simulink model "untitled"  (R2026a)
settings: Solver=FixedStepDiscrete  StartTime=0  StopTime=0.2  FixedStep=5e-05
settings Model: Creator=nairizeytounzian  LastModifiedBy=nairizeytounzian

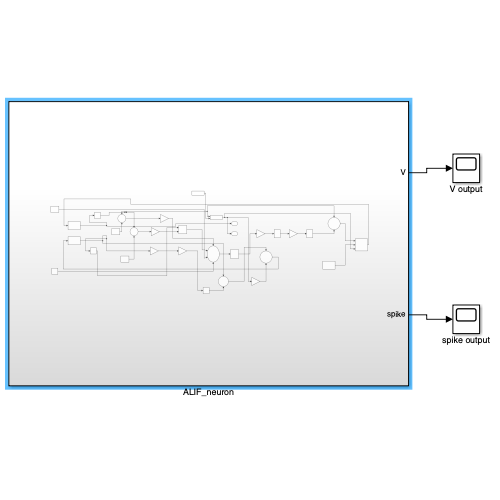
[thumbnail: Simulink's stored preview of the top-level diagram]
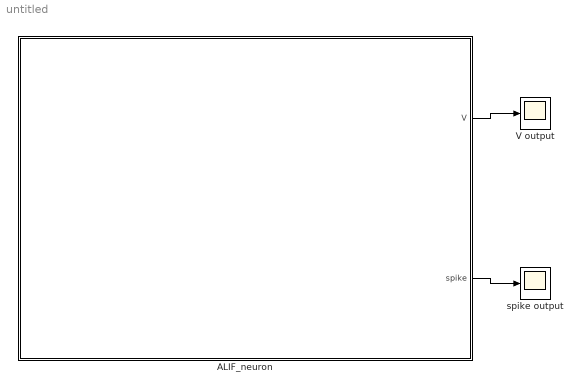
== system untitled ==
  ALIF_neuron : Subsystem
  V output : Scope
      settings: ActiveDisplayYMinimum=-74.012180112119538  ActiveDisplayYMaximum=-48.080272939355147
  spike output : Scope
      settings: ActiveDisplayYMinimum=-0.12499999999999997  ActiveDisplayYMaximum=1.125
  wires:
  ALIF_neuron/1(V) -> V output/1
  ALIF_neuron/2(spike) -> spike output/1

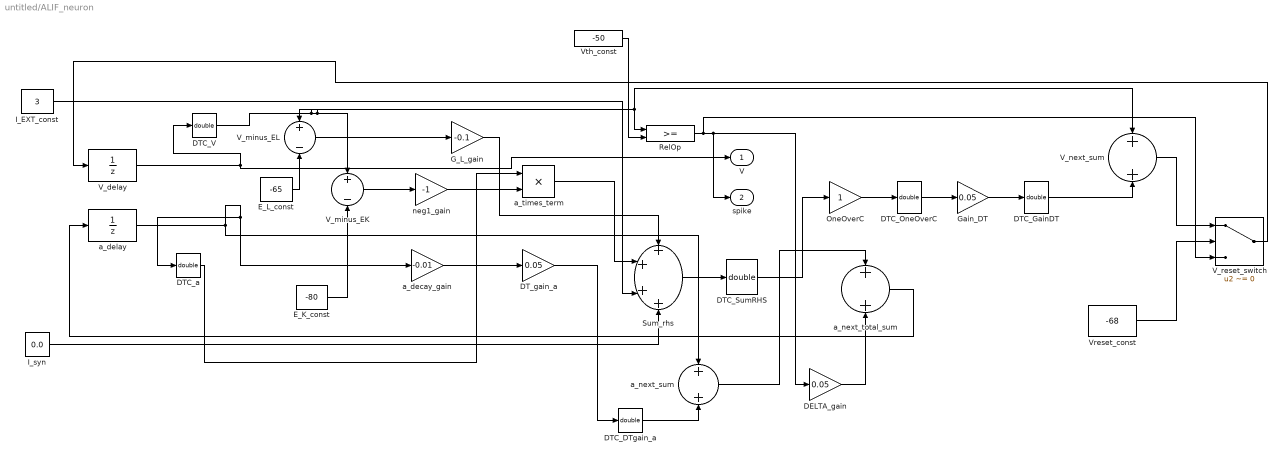
== system untitled/ALIF_neuron ==
  DELTA_gain : Gain  Gain=0.05
  DTC_DTgain_a : DataTypeConversion  OutDataTypeStr=double  SaturateOnIntegerOverflow=off  RndMeth=Floor
  DTC_GainDT : DataTypeConversion  OutDataTypeStr=double  SaturateOnIntegerOverflow=off  RndMeth=Floor
  DTC_OneOverC : DataTypeConversion  OutDataTypeStr=double  SaturateOnIntegerOverflow=off  RndMeth=Floor
  DTC_SumRHS : DataTypeConversion  OutDataTypeStr=double  SaturateOnIntegerOverflow=off  RndMeth=Floor
  DTC_V : DataTypeConversion  OutDataTypeStr=double  SaturateOnIntegerOverflow=off  RndMeth=Floor
  DTC_a : DataTypeConversion  OutDataTypeStr=double  SaturateOnIntegerOverflow=off  RndMeth=Floor
  DT_gain_a : Gain  Gain=0.05
  E_K_const : Constant  Value=-80  OutDataTypeStr=double
  E_L_const : Constant  Value=-65  OutDataTypeStr=double
  G_L_gain : Gain  Gain=-0.1
  Gain_DT : Gain  Gain=0.05
  I_EXT_const : Constant  Value=3  OutDataTypeStr=double
  I_syn : Constant  Value=0.0
  OneOverC : Gain
  RelOp : RelationalOperator  OutDataTypeStr=boolean  RndMeth=Simplest  InputSameDT=off
  Sum_rhs : Sum  Inputs=++++
  V_delay : UnitDelay  InitialCondition=-65  SampleTime=-1
  V_minus_EK : Sum  Inputs=+-
  V_minus_EL : Sum  Inputs=+-
  V_next_sum : Sum
  V_reset_switch : Switch  Criteria=u2 ~= 0  Threshold=0.5  SaturateOnIntegerOverflow=off  InputSameDT=off
  Vreset_const : Constant  Value=-68  OutDataTypeStr=double
  Vth_const : Constant  Value=-50  OutDataTypeStr=double
  a_decay_gain : Gain  Gain=-0.01
  a_delay : UnitDelay  SampleTime=-1
  a_next_sum : Sum
  a_next_total_sum : Sum
  a_times_term : Product
  neg1_gain : Gain  Gain=-1
  V : Outport
  spike : Outport  Port=2
  wires:
  V_delay/1 -> DTC_V/1, V/1
  DTC_V/1 -> V_minus_EK/1, V_minus_EL/1, V_next_sum/1, RelOp/1
  E_L_const/1 -> V_minus_EL/2
  E_K_const/1 -> V_minus_EK/2
  V_minus_EL/1 -> G_L_gain/1
  G_L_gain/1 -> Sum_rhs/1
  V_minus_EK/1 -> neg1_gain/1
  neg1_gain/1 -> a_times_term/2
  a_delay/1 -> DTC_a/1, a_decay_gain/1, a_next_sum/1
  DTC_a/1 -> a_times_term/1
  a_times_term/1 -> Sum_rhs/2
  I_EXT_const/1 -> Sum_rhs/3
  I_syn/1 -> Sum_rhs/4
  Sum_rhs/1 -> DTC_SumRHS/1
  DTC_SumRHS/1 -> OneOverC/1
  OneOverC/1 -> DTC_OneOverC/1
  DTC_OneOverC/1 -> Gain_DT/1
  Gain_DT/1 -> DTC_GainDT/1
  DTC_GainDT/1 -> V_next_sum/2
  V_next_sum/1 -> V_reset_switch/1
  Vreset_const/1 -> V_reset_switch/2
  Vth_const/1 -> RelOp/2
  RelOp/1 -> spike/1, DELTA_gain/1, V_reset_switch/3
  V_reset_switch/1 -> V_delay/1
  a_decay_gain/1 -> DT_gain_a/1
  DT_gain_a/1 -> DTC_DTgain_a/1
  DTC_DTgain_a/1 -> a_next_sum/2
  a_next_sum/1 -> a_next_total_sum/1
  DELTA_gain/1 -> a_next_total_sum/2
  a_next_total_sum/1 -> a_delay/1
